simulink model "SignalMesurement"  (R2023b)
settings: Solver=VariableStepAuto  StartTime=0.0  StopTime=2  RelTol=1e-3
libraries: fl_lib x6, nesl_utility x3, spspowerguiLib x1
settings Model: Creator=Admin  LastModifiedBy=Admin
settings DebuggingCC: ParameterPrecisionLossMsg=none

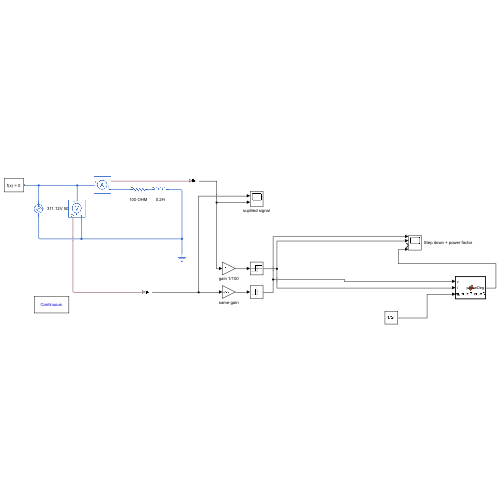
[thumbnail: Simulink's stored preview of the top-level diagram]
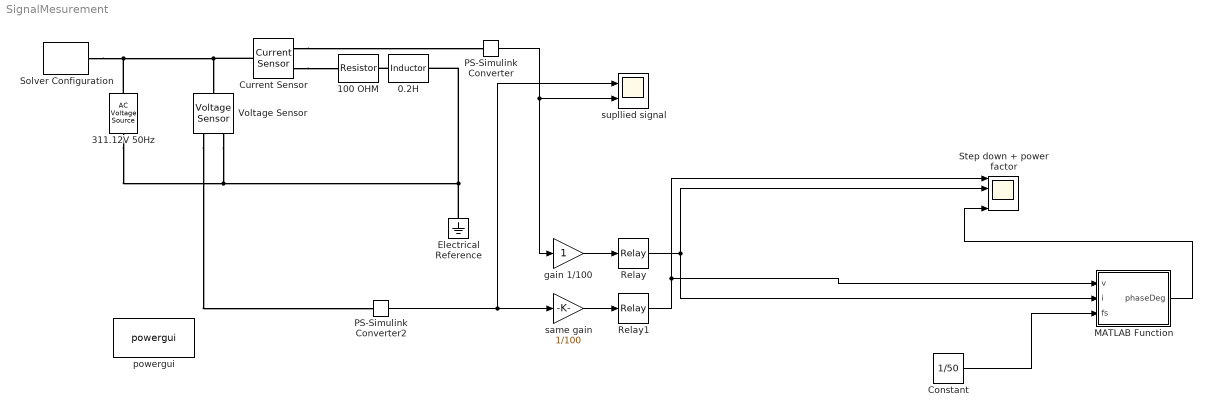
== system SignalMesurement ==
  0.2H : fl_lib/Electrical/Electrical Elements/Inductor  l=0.2 H  r=0 Ohm  g=1e-9 1/Ohm  i_specify=off  i_priority=None  i=0 A  i_nominal_specify=off  i_nominal_unit=A  i_nominal_value=1  v_specify=off  v_priority=None  v=0 V  v_nominal_specify=off  v_nominal_unit=V  v_nominal_value=1  i_L_specify=off  i_L_priority=High  i_L=0 A  i_L_nominal_specify=off  i_L_nominal_unit=A  i_L_nominal_value=1
  "100 OHM " : fl_lib/Electrical/Electrical Elements/Resistor  R=100 Ohm  i_specify=off  i_priority=None  i=0 A  i_nominal_specify=off  i_nominal_unit=A  i_nominal_value=1  v_specify=off  v_priority=None  v=0 V  v_nominal_specify=off  v_nominal_unit=V  v_nominal_value=1
  311.12V 50Hz : fl_lib/Electrical/Electrical Sources/AC Voltage Source  amp=311.12 V  shift=0 deg  frequency=50 Hz  omega=0 rad/s
  Constant : Constant  Value=1/50
  Current Sensor : fl_lib/Electrical/Electrical Sensors/Current Sensor
  Electrical Reference : fl_lib/Electrical/Electrical Elements/Electrical Reference
  MATLAB Function : MATLAB Function  TreatAsAtomicUnit=on
  PS-Simulink Converter : nesl_utility/PS-Simulink Converter  PhysicalDomain=network_engine_domain  SubClassName=ps_output  LeftPortType=input  RightPortType=output  PseudoPeriodic=off  Frequencies=[]  VectorFormat=inherit  Unit=inherit  AffineConversion=off
  PS-Simulink Converter2 : nesl_utility/PS-Simulink Converter  PhysicalDomain=network_engine_domain  SubClassName=ps_output  LeftPortType=input  RightPortType=output  PseudoPeriodic=off  Frequencies=[]  VectorFormat=inherit  Unit=inherit  AffineConversion=off
  Relay : Relay  OnSwitchValue=0.05  OffSwitchValue=-0.05  OutDataTypeStr=double
  Relay1 : Relay  OnSwitchValue=0.05  OffSwitchValue=-0.05  OutDataTypeStr=boolean
  Solver Configuration : nesl_utility/Solver Configuration  PhysicalDomain=network_engine_domain  SubClassName=solver  LeftPortType=input  RightPortType=generic  Tones=[]  Harmonics=[]  SimulateNoise=off  Profile=off  UseLocalSampling=off  EnableSwitchedLinearOptims=on  FrequencyDomain=off  UseCCode=off  RelTol=0.001  AbsTol=0.001  MinStep=1e-09  ToWorkspace=off  RevertToSquareIcSolve=off  NumHomotopyIterations=100  PhasorMode=off  PhasorModeNumHarmonics=1  ConsistencySolver=NEWTON_XTOL_AFTER_FTOL  IndexReductionMethod=DerivativeReplacement  DoDC=off  ResidualTolerance=1e-09  ConsistencyTolSource=GLOBAL  ConsistencyAbsTol=0.001  ConsistencyRelTol=0.001  ConsistencyTolFactor=0.001  UseLocalSolver=off  LocalSolverChoice=NE_BACKWARD_EULER_ADVANCER  ResolveIndetEquations=on  FunctionEvalNumThread=1  LocalSolverSampleTime=0.001  DoFixedCost=off  MaxNonlinIter=3  MaxModeIter=2  ComputeImpulses=off  ImpulseIterations=2  LinearAlgebra=auto  LinearAlgebraNumThread=0  EquationFormulation=NE_TIME_EF  DelaysMemoryBudget=1024  AutomaticFiltering=on  FilteringTimeConstant=0.001  PartitionStorageMethod=AS_NEEDED  PartitionMemoryBudget=1024  PartitionMethod=ROBUST  MultibodyUseLocalSolver=off  MultibodyLocalSolverChoice=ODE1  MultibodyLocalSolverSampleTime=0.001
  Step down + power factor : Scope  NumInputPorts=4
  Voltage Sensor : fl_lib/Electrical/Electrical Sensors/Voltage Sensor
  gain 1/100 : Gain
  powergui : spspowerguiLib/powergui  Priority=1  SimulationMode=Continuous  SampleTime=50e-6  frequency=60  Iterations=50  frequencyindice=60  Pbase=100e6  ErrMax=1e-4  UnitsV=kV  UnitsW=MW  buscounter=0  FunctionMessages=off  echomessages=off  EnableUseOfTLC=off  CurrentSourceSwitches=off  DisableSnubberDevices=off  DisableRonSwitches=off  DisableVfSwitches=off  DisplayEquations=off  AutomaticDiscreteSolvers=off  SolverType=Tustin/Backward Euler (TBE)  Interpol=off  ExternalGateDelay=off  methode=off  Ts=100  x0status=blocks  SPID=on  SwTol=0  HookPort=off  NonlinearTolerance=1e-4  nMaxIteration=100  ContinueOnMaxIteration=off  RestoreLinks=warning  ResistiveCurrentMeasurement=off  Frange=[0:2:500]  Ylog=off  Xlog=on  ShowGrid=off  save=off  variable=ZData  structure=0  ZoomFFT=off  StartTime=0.0  cycles=1  DisplayStyle=1  fundamental=60  FreqAxis=off  MaxFrequency=1000  frequencyindicesteady=1  RmsSteady=1  display=off
  same gain : Gain  Gain=1/100  OutDataTypeStr=double
  supllied signal : Scope  NumInputPorts=2
  wires:
  gain 1/100/1 -> Relay/1
  same gain/1 -> Relay1/1
  Relay/1 -> Step down + power factor/2, MATLAB Function/2(i)
  Relay1/1 -> MATLAB Function/1(v), Step down + power factor/1
  PS-Simulink Converter2/1 -> supllied signal/1, same gain/1
  PS-Simulink Converter/1 -> gain 1/100/1, supllied signal/2
  MATLAB Function/1(phaseDeg) -> Step down + power factor/4
  Constant/1 -> MATLAB Function/3(fs)
  connections:
  0.2H/LConn1 -- "100 OHM "/RConn1
  Current Sensor/RConn2 -- "100 OHM "/LConn1
  Voltage Sensor/RConn2 -- Electrical Reference/LConn1 -- 0.2H/RConn1 -- 311.12V 50Hz/RConn1
  Voltage Sensor/RConn1 -- PS-Simulink Converter2/LConn1
  Current Sensor/RConn1 -- PS-Simulink Converter/LConn1
  Solver Configuration/RConn1 -- 311.12V 50Hz/LConn1 -- Current Sensor/LConn1 -- Voltage Sensor/LConn1

== matlab function SignalMesurement/MATLAB Function ==
  data: v input; i input; phaseDeg output; fs input
function phaseDeg = measurePhaseDiff(v, i, fs)
    % v  : Voltage vector
    % i  : Current vector
    % fs : Sampling frequency (Hz)
    
    % Ensure signals are zero-centered (remove DC offset)
    v = v - mean(v);
    i = i - mean(i);
    
    % Use Hilbert Transform to get the analytic signal
    analytic_v = hilbert(v);
    analytic_i = hilbert(i);
    
    % Calculate the instantaneous phase of each signal
    phase_v = angle(analytic_v);
    phase_i = angle(analytic_i);
    
    % The difference in phase (wrapped between -pi and pi)
    % We take the mean difference across the steady-state portion
    phaseDiffRad = mean(angle(exp(1i * (phase_v - phase_i))));
    
    % Convert to degrees
    phaseDeg = rad2deg(phaseDiffRad);
end
